simulink model "controlSystem"  (R2013b)
settings: Solver=ode1  StartTime=0.0  StopTime=tSim  FixedStep=0.1  RelTol=1e-3
values from neighbouring files (symbols this model uses):
  initial_state = -1    [launcher.m]
  input = 1    [launcher.m]
  k = 4    [launcher.m]
  P = 2    [launcher.m]
  switch_time = 2    [launcher.m]
  T = 3    [launcher.m]
settings Model: Creator=JT  LastModifiedBy=JT

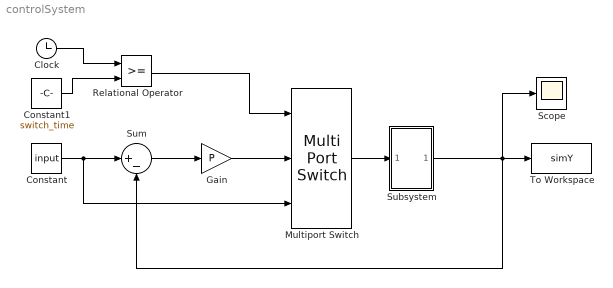
== system controlSystem ==
  Clock : Clock
  Constant : Constant  Value=input
  Constant1 : Constant  Value=switch_time
  Gain : Gain  Gain=P
  Multiport Switch : MultiPortSwitch  DataPortOrder=Zero-based contiguous  Inputs=2
  Relational Operator : RelationalOperator  OutDataTypeStr=boolean
  Scope : Scope
  Subsystem : Subsystem
  Sum : Sum  Inputs=|+-
  To Workspace : ToWorkspace  VariableName=simY  SampleTime=-1
  wires:
  Constant/1 -> Multiport Switch/3, Sum/1
  Sum/1 -> Gain/1
  Clock/1 -> Relational Operator/1
  Constant1/1 -> Relational Operator/2
  Multiport Switch/1 -> Subsystem/1(In1)
  Relational Operator/1 -> Multiport Switch/1
  Gain/1 -> Multiport Switch/2
  Subsystem/1(Out1) -> Sum/2, Scope/1, To Workspace/1

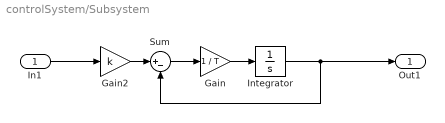
== system controlSystem/Subsystem ==
  In1 : Inport
  Gain : Gain  Gain=1 / T
  Gain2 : Gain  Gain=k
  Integrator : Integrator  InitialCondition=initial_state
  Sum : Sum  Inputs=|+-
  Out1 : Outport
  wires:
  Sum/1 -> Gain/1
  Integrator/1 -> Out1/1, Sum/2
  Gain2/1 -> Sum/1
  In1/1 -> Gain2/1
  Gain/1 -> Integrator/1
